simulink model "simple_FXTDiff_ANSFT"  (R2024b)
settings: Solver=ode4  StartTime=0.0  StopTime=15  FixedStep=0.01  RelTol=1e-3
model workspace (MAT data in the model file):
  roll = [0 0.5 0 -0.5 0 0.5]
  tra1 = [0 2 0 -2 0 2]
  tra2 = [0 2 2 2 2 0]
  tra3 = [0 0 2 2 2 2]
values from neighbouring files (symbols this model uses):
  F = 5    [assignment3.m]
undefined symbols (not defined in the file or in its folder): Light, MIL
libraries: dspobslib x7, simulink x5, robotcorelib x1, aerolibwind2 x1
settings Model: Creator=Adan Daniel  LastModifiedBy=danyy
settings OptimizationCC: ReuseModelBlockBuffer=off
settings RTWCC: GPUComputeCapability=3.5

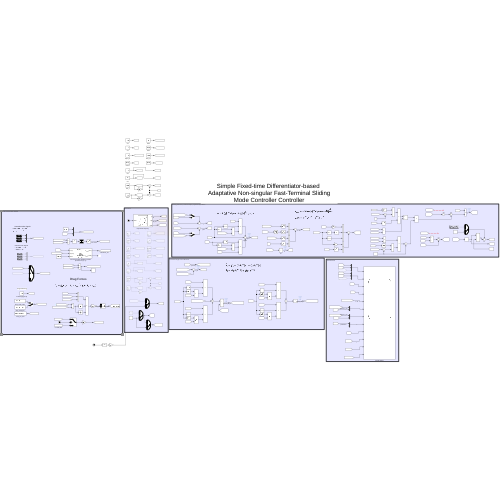
[thumbnail: Simulink's stored preview of the top-level diagram]
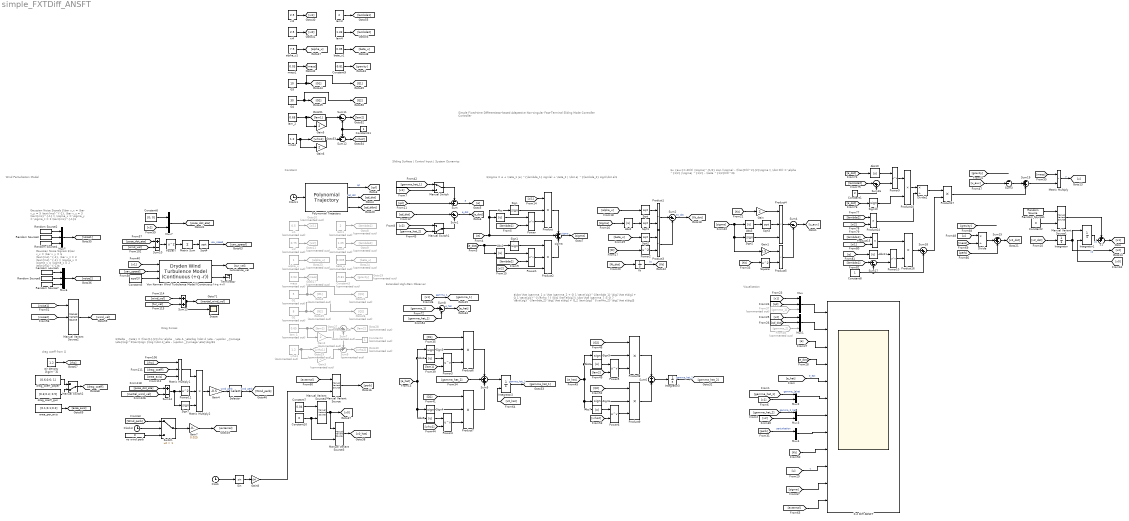
== system simple_FXTDiff_ANSFT ==
  note: Wind Perturbation Model
  note: Extended High-Gain Observer
  note: Sliding Surface | Control Input | System Dynamics
  note: Constant
  note: Visualization
  note: Simple Fixed-time Differentiator-based
      | Adaptative Non-singular Fast-Terminal Sliding Mode Controller Controller
  note: $\sigma = e + \zeta_1 |e| ^{\lambda_1} sign(e) + \zeta_2 | \dot e| ^{\lambda_2} sign(\dot e)$
  note: $u_{aux}=-2K(t) |\sigma|^{1/2} sign (\sigma) - \frac{K(t)^2}{2}\sigma \\ \dot K(t) = \alpha ^{1/2} |\sigma| ^{1/2} - \beta ^{1/2}K(t)^2$
  note: $\dot \hat \gamma_1 = \hat \gamma_2 + G_1 \text{sig}^{\lambda_1} \big[ \hat e\big] + Q_1 \text{sig}^{\varrho_1} \big[ \hat e\big] \\ \dot \hat \gamma_2 = G_2 \text{sig}^{\lambda_2} \big[ \hat e\big] + Q_2 \text{sig}^{\varrho_2} \big[ \hat e\big]$
  note: Gaussian Noise Signals
      | $\bar v_x = \bar v_y = 5 \text{ms}^{-1}, \bar v_z = 3 \text{ms}^{-1} \\ \sigma_x = \sigma_y = \sigma_z = 2 \text{ms}^{-1}$
  note: Gaussian Noise Signals
      | $\bar v_x = \bar v_y = 6 \text{ms}^{-1}, \bar v_z = 2 \text{ms}^{-1} \\ \sigma_x = \sigma_y = \sigma_z = 2 \text{ms}^{-1}$
  note: Drag Forces
  note: $\Delta _ {\eta} = \frac{1}{2}\rho \alpha _ \eta A _\eta\big (\dot d_\eta - \upsilon _{\omega \eta}\big)^2\text{sign }\big (\dot d_\eta - \upsilon _{\omega \eta}\big)$$
  note: drag coeff from []
  Abs{,1..7,10..11} (10 alike) : Abs  SaturateOnIntegerOverflow=off
  Clock : Clock
  Clock1 : Clock
  Clock3 : Clock
  Constant1 : Constant  Value=2
  Constant10 : Constant  Value=0
  Constant11 : Constant
  Constant2 : Constant  Value=0
  Constant3 : Constant  Commented=on  Value=-9.81
  Constant4 : Constant  Commented=on
  Constant5 : Constant  Value=eye(3)
  Constant6 : Constant  Value=[0; 0]
  Constant7 : Constant  Value=0.04
  Constant8 : Constant
  Constant9 : Constant  Value=-9.81
  Divide : Product  Inputs=*/
  Divide2 : Product  Inputs=*/
  From37 : From  Commented=on  GotoTag=gamma_1
  From38 : From  Commented=on  GotoTag=gamma_2
  Fxt Diff ANSFT : Scope  NumInputPorts=12
  G1 : Constant  Commented=on  Value=5
  G2 : Constant  Commented=on  Value=8
  G3 : Constant  Value=10
  G4 : Constant  Value=30
  Gain : Gain  Gain=2
  Gain1 : Gain  Gain=0.5
  Gain2 : Gain  Commented=on  Gain=2
  Gain3 : Gain  Commented=on  Gain=2
  Gain4 : Gain  Gain=-0.5
  Gain5 : Gain  Gain=2
  Gain6 : Gain  Gain=2
  Gain7 : Gain  Gain=0.025
  Gain8 : Gain  Gain=0.04
  Goto10 : Goto  Commented=on  GotoTag=xi1
  Goto11 : Goto  Commented=on  GotoTag=xi2
  Goto17 : Goto  Commented=on  GotoTag=mass
  Goto19 : Goto  Commented=on  GotoTag=gravity
  Goto2 : Goto  Commented=on  GotoTag=G1
  Goto22 : Goto  Commented=on  GotoTag=Q1
  Goto23 : Goto  Commented=on  GotoTag=alpha_u
  Goto24 : Goto  Commented=on  GotoTag=beta_u
  Goto25 : Goto  Commented=on  GotoTag=G2
  Goto26 : Goto  Commented=on  GotoTag=Q2
  Goto27 : Goto  Commented=on  GotoTag=lam1
  Goto28 : Goto  Commented=on  GotoTag=lam2
  Goto29 : Goto  Commented=on  GotoTag=vrho1
  Goto30 : Goto  Commented=on  GotoTag=vrho2
  Goto8 : Goto  Commented=on  GotoTag=lambda1
  Goto9 : Goto  Commented=on  GotoTag=lambda2
  Integrator : Integrator
  Integrator1 : Integrator  InitialConditionSource=external
  Integrator2 : Integrator  InitialConditionSource=external
  Integrator3 : Integrator
  Kt : Integrator
  Manual Variant Source{,1,3..4} (4 alike) : simulink/Signal Routing/Manual Variant Source  NumChoices=2  LabelModeActiveChoice=V_2
  Manual Variant Source2 : simulink/Signal Routing/Manual Variant Source  NumChoices=3  LabelModeActiveChoice=V_1
  Manual Switch : ManualSwitch
  Manual Switch1 : ManualSwitch  CurrentSetting=0
  Manual Switch2 : ManualSwitch  CurrentSetting=0
  Matrix Sum : Sum  Inputs=+
  Matrix Multiply : Product
  Matrix Multiply1 : Product  Inputs=3
  Matrix Multiply2 : Product  Inputs=3
  Mux{,1,5..6} (4 alike) : Mux  Inputs=3
  Mux{2..4,7} (4 alike) : Mux  Inputs=2
  Polynomial Trajectory : robotcorelib/Polynomial Trajectory  WaypointSource=Internal  Waypoints=[0, 0, 0.15, -0.15, 0.1, -0.1]*0  TimePoints=[0, 5, 10, 15, 20, 25]/5  TimeInterval=[ 1, 4 ]  Method=Cubic Polynomial  ParameterSource=Internal  VelocityBoundaryCondition=zeros( 1, 6 )  AccelerationBoundaryCondition=zeros( 2, 5 )  SimulateUsing=Interpreted execution
  Power{,1,3..6,9..10} (8 alike) : Math  Operator=pow
  Power11 : Math  Operator=square
  Power2 : Math  Operator=square
  Power7 : Math  Operator=square
  Product{,2,4,6..9} (7 alike) : Product  Inputs=3
  Product{1,3,5,10,14..17} (8 alike) : Product
  Random Source1 : dspobslib/Random Source  SrcType=Gaussian  NormMethod=Ziggurat  CltLength=12  MinVal=0  MaxVal=1  MeanVal=0.005  VarVal=0.001 * 0.001  RepMode=Repeatable  rawSeed=1  IsInherit=off  SampMode=Continuous  SampTime=0.01  SampFrame=1  DataType=Double  OutComplex=Real  OutputFrames=off
  Random Source2 : dspobslib/Random Source  SrcType=Gaussian  NormMethod=Ziggurat  CltLength=12  MinVal=0  MaxVal=1  MeanVal=5  VarVal=2  RepMode=Not repeatable  rawSeed=1  IsInherit=off  SampMode=Discrete  SampTime=1  SampFrame=1  DataType=Double  OutComplex=Real  OutputFrames=off
  Random Source3 : dspobslib/Random Source  SrcType=Gaussian  NormMethod=Ziggurat  CltLength=12  MinVal=0  MaxVal=1  MeanVal=5  VarVal=2  RepMode=Not repeatable  rawSeed=1  IsInherit=off  SampMode=Discrete  SampTime=1  SampFrame=1  DataType=Double  OutComplex=Real  OutputFrames=off
  Random Source4 : dspobslib/Random Source  SrcType=Gaussian  NormMethod=Ziggurat  CltLength=12  MinVal=0  MaxVal=1  MeanVal=3  VarVal=2  RepMode=Not repeatable  rawSeed=1  IsInherit=off  SampMode=Discrete  SampTime=1  SampFrame=1  DataType=Double  OutComplex=Real  OutputFrames=off
  Random Source5 : dspobslib/Random Source  SrcType=Gaussian  NormMethod=Ziggurat  CltLength=12  MinVal=0  MaxVal=1  MeanVal=6  VarVal=2  RepMode=Not repeatable  rawSeed=1  IsInherit=off  SampMode=Discrete  SampTime=1  SampFrame=1  DataType=Double  OutComplex=Real  OutputFrames=off
  Random Source6 : dspobslib/Random Source  SrcType=Gaussian  NormMethod=Ziggurat  CltLength=12  MinVal=0  MaxVal=1  MeanVal=6  VarVal=2  RepMode=Not repeatable  rawSeed=1  IsInherit=off  SampMode=Discrete  SampTime=1  SampFrame=1  DataType=Double  OutComplex=Real  OutputFrames=off
  Random Source7 : dspobslib/Random Source  SrcType=Gaussian  NormMethod=Ziggurat  CltLength=12  MinVal=0  MaxVal=1  MeanVal=2  VarVal=2  RepMode=Not repeatable  rawSeed=1  IsInherit=off  SampMode=Discrete  SampTime=1  SampFrame=1  DataType=Double  OutComplex=Real  OutputFrames=off
  Scope : Scope
  Selector : Selector  InputPortWidth=3  IndexOptions=Index vector (dialog)  Indices=[3]  OutputSizes=1
  Sign{,1..7,10} (9 alike) : Signum
  Sin : Trigonometry
  Sqrt{,1..4} (5 alike) : Sqrt
  Square : Math  Operator=square
  Sum : Sum  Inputs=-+|
  Sum{1..2,8,11,17} (5 alike) : Sum  Inputs=|+-
  Sum10 : Sum  Inputs=+-
  Sum12 : Sum  Inputs=-+|
  Sum13 : Sum
  Sum14 : Sum  Inputs=+-
  Sum15 : Sum  Inputs=+++
  Sum16 : Sum  Inputs=|-+
  Sum18 : Sum  Inputs=|++
  Sum19 : Sum  Inputs=+++
  Sum3 : Sum  Inputs=--|
  Sum4 : Sum  Inputs=|--
  Sum5 : Sum  Inputs=+++
  Sum6 : Sum  Inputs=+|+
  Sum7 : Sum  Commented=on  Inputs=|+-
  Sum9 : Sum  Commented=on  Inputs=-+|
  Switch : Switch  Criteria=u2 > Threshold  Threshold=1  SaturateOnIntegerOverflow=off  InputSameDT=off
  Terminator : Terminator
  Von Karman Wind Turbulence Model (Continuous (+q +r)) : aerolibwind2/Dryden Wind Turbulence Model  (Continuous (+q -r))  units=Metric (MKS)  spec=MIL-F-8785C  model=Continuous Von Karman (+q +r)  W20=15  Wdeg=0  TurbProb=10^-2 - Light  L_high=762  Wingspan=10  ts=0.1  Seed=[23341 23342 23343 23344]  T_on=on
      settings: LibrarySourceBlock=|
      | aerolibwind2/Von Karman Wind Turbulence Model
      | (Continuous (+q +r))
  air density [kg/m^3] : Constant  Value=1.2
  alpha_u : Constant  Commented=on
  alpha_u1 : Constant  Value=7.5
  area_per_axis : Constant  Value=[0.1;0.1;0.2]
  beta_u : Constant  Commented=on  Value=0.005
  beta_u1 : Constant  Value=0.05
  drag_coeff_gus : Constant  Value=[0.3;0.3; 0.5]
  drag_coeff_paper : Constant  Value=[0.6;0.6; 1]
  lam1 : Constant  Commented=on  Value=2
  lam2 : Constant  Commented=on  Value=1.25
  lam3 : Constant  Value=2
  lam4 : Constant  Value=1.33
  lam_1 : Constant  Commented=on  Value=0.65
  lam_2 : Constant  Value=0.68
  mass : Constant  Commented=on  Value=0.03
  mass1 : Constant  Value=0.03
  no wind perb : Constant  Value=0
  sigma : Sum  Inputs=+++
  vrho1 : Constant  Commented=on  Value=1.2
  vrho2 : Constant  Value=1.2
  x1 : Sum  Inputs=++|
  xi1 : Constant  Commented=on  Value=0.5
  xi2 : Constant  Commented=on  Value=0.75
  xi3 : Constant  Value=2.5
  xi4 : Constant  Value=2.5
  wires:
  Integrator/1 -> [x2], Integrator1/1  "x2"
  Sum1/1 -> [e_dot]  "e_dot"
  Mux/1 -> Fxt Diff ANSFT/1
  [x2_dot] -> Integrator/1
  Clock1/1 -> Polynomial Trajectory/1
  Polynomial Trajectory/3 -> [qd_ddot]
  [gamma_1] -> Sum8/1
  [gamma_hat_1] -> Sum8/2
  Sum8/1 -> [e_hat]  "e_hat"
  [e_hat] -> Fxt Diff ANSFT/5  "e_est"
  [gamma_hat_1] -> Mux2/1  "gamma_1_hat"
  [gamma_hat_2] -> Mux3/1  "gamma_2_hat"
  Mux2/1 -> Fxt Diff ANSFT/6
  [x1] -> Mux2/2
  Mux3/1 -> Fxt Diff ANSFT/7
  [x1] -> Manual Switch/2
  [x2] -> Manual Switch1/1
  [qd] -> Mux/2
  Polynomial Trajectory/1 -> [qd]  "qd"
  Polynomial Trajectory/2 -> [qd_dot]  "qd_dot"
  [qd] -> Sum/2
  [qd_dot] -> Sum1/1
  Sum/1 -> [e]  "e"
  lam1/1 -> Goto8/1
  lam2/1 -> Goto9/1
  xi1/1 -> Goto10/1
  xi2/1 -> Goto11/1
  [x1] -> Mux/1
  [qd_dot] -> Mux1/2
  [x2] -> Mux1/1
  Mux1/1 -> Fxt Diff ANSFT/2
  [e] -> Fxt Diff ANSFT/3
  [e_dot] -> Fxt Diff ANSFT/4
  [x1] -> [gamma_1]  "gamma_1"
  [x2] -> Mux3/2
  [perb] -> Mux4/1  "perturbation"
  Manual Variant Source/1 -> [perb]
  Mux4/1 -> Fxt Diff ANSFT/8
  mass/1 -> Goto17/1
  From37/1 -> Mux/3
  From38/1 -> Mux1/3
  Manual Switch/1 -> Sum/1
  Manual Switch1/1 -> Sum1/2
  [gamma_hat_2] -> Manual Switch1/2
  [gamma_hat_1] -> Manual Switch/1
  Constant3/1 -> Goto19/1
  [Kt] -> Fxt Diff ANSFT/9
  [u] -> Fxt Diff ANSFT/10  "u"
  [u] -> Divide/1
  [e] -> sigma/2, Abs/1, Sign/1
  Abs/1 -> Power/1
  [lambda1] -> Power/2
  Power/1 -> Product/3
  Sign/1 -> Product/2
  sigma/1 -> [sigma]  "sigma"
  Power1/1 -> Product2/2
  [e_dot] -> Abs1/1, Sign1/1
  [lambda2] -> Power1/2
  Abs1/1 -> Power1/1
  Sign1/1 -> Product2/1
  Product2/1 -> sigma/3
  Product/1 -> sigma/1
  [xi1] -> Product/1
  [xi2] -> Product2/3
  beta_u/1 -> Goto24/1
  alpha_u/1 -> Goto23/1
  [Kt] -> Power2/1
  [alpha_u] -> Sqrt/1
  [sigma] -> Abs2/1
  Abs2/1 -> Sqrt1/1
  Sqrt1/1 -> Product1/2
  Power2/1 -> Product3/2
  [beta_u] -> Sqrt2/1
  Sqrt/1 -> Product1/1
  Product3/1 -> Sum2/2
  Product1/1 -> Sum2/1
  Sqrt2/1 -> Product3/1
  Sum2/1 -> [Kt_dot]  "Kt_dot"
  [Kt_dot] -> Kt/1
  Kt/1 -> [Kt]  "kt"
  Sqrt3/1 -> Product4/2
  Product4/1 -> Sum4/1
  Abs3/1 -> Sqrt3/1
  [sigma] -> Abs3/1, Sign2/1, Gain1/1
  Gain/1 -> Product4/1
  [Kt] -> Gain/1
  Sign2/1 -> Product4/3
  [Kt] -> Square/1
  Square/1 -> Product5/2
  Gain1/1 -> Product5/1
  Product5/1 -> Sum4/2
  Sum4/1 -> [u_aux]
  Matrix Multiply/1 -> [u]  "u"
  Sum15/1 -> [x2_dot]
  [sigma] -> Fxt Diff ANSFT/11
  [mass] -> Divide/2
  Divide/1 -> Sum15/2
  [perb] -> Sum15/3
  [gravity] -> ?
  [mass] -> Matrix Multiply/1
  [u_aux] -> Sum3/2
  [e_dot] -> Abs10/1
  Sum16/1 -> Power9/2
  Sign10/1 -> Product10/2
  Abs10/1 -> Power9/1
  Product14/1 -> Divide2/2
  Constant1/1 -> Sum16/2
  [lambda2] -> Sum16/1
  Power9/1 -> Product10/1
  [lambda2] -> Product14/1
  [e_dot] -> Sign10/1
  Product10/1 -> Divide2/1
  [xi2] -> Product14/2
  Product15/1 -> Product16/1
  Product16/1 -> Sum18/1
  Power10/1 -> Product16/2
  Constant8/1 -> Sum18/2, Sum17/2
  [xi1] -> Product15/2
  [lambda1] -> Product15/1
  Abs11/1 -> Power10/1
  [lambda1] -> Sum17/1
  [e] -> Abs11/1
  Sum17/1 -> Power10/2
  Divide2/1 -> Product17/1
  Sum18/1 -> Product17/2
  Sum19/1 -> Matrix Multiply/2
  Sum3/1 -> Sum19/2
  Product17/1 -> Sum19/3
  Sum5/1 -> Integrator2/1
  Sign6/1 -> Product9/2
  Power5/1 -> Product8/3
  Power6/1 -> Product9/3
  [Q2] -> Product9/1
  [G2] -> Product8/1
  Power4/1 -> Product7/3
  [vrho2] -> Power6/2
  Sign5/1 -> Product8/2
  Product7/1 -> Sum5/3
  [Q1] -> Product7/1
  Integrator3/1 -> [gamma_hat_2]  "gamma_hat_2"
  Product8/1 -> Sum6/1
  [gamma_hat_2] -> Sum5/2
  [lam2] -> Power5/2
  [lam1] -> Power3/2
  Abs4/1 -> Power3/1
  Power3/1 -> Product6/3
  [e_hat] -> Sign3/1, Abs4/1, Abs5/1, Sign4/1
  [G1] -> Product6/1
  Integrator2/1 -> [gamma_hat_1]  "gamma_hat_1"
  Product6/1 -> Sum5/1
  Abs7/1 -> Power6/1
  Sign4/1 -> Product7/2
  Abs5/1 -> Power4/1
  Abs6/1 -> Power5/1
  [vrho1] -> Power4/2
  Product9/1 -> Sum6/2
  Sign3/1 -> Product6/2
  Sum6/1 -> Integrator3/1
  [e_hat] -> Sign5/1, Abs6/1, Abs7/1, Sign6/1
  G2/1 -> Goto26/1, Goto25/1
  lam_1/1 -> Gain2/1, Goto27/1
  vrho1/1 -> Gain3/1, Goto29/1
  G1/1 -> Goto22/1, Goto2/1
  [gravity] -> ?
  Constant2/1 -> Manual Variant Source1/2
  Random Source1/1 -> Manual Variant Source1/1
  Integrator1/1 -> x1/2  "x1"
  x1/1 -> [x1]
  Manual Variant Source1/1 -> x1/1
  Gain2/1 -> Sum7/1
  Sum7/1 -> Goto28/1
  Constant4/1 -> Sum7/2, Sum9/1
  Gain3/1 -> Sum9/2
  Sum9/1 -> Goto30/1
  Constant5/1 -> Von Karman Wind Turbulence Model (Continuous (+q +r))/3
  [x1] -> Von Karman Wind Turbulence Model (Continuous (+q +r))/1
  Von Karman Wind Turbulence Model (Continuous (+q +r))/1 -> [tur_vel]
  [tur_vel] -> Sum13/2
  Sum13/1 -> Scope/1, [inertial_wind_vel]
  [wind_vel] -> Sum13/1
  Random Source4/1 -> Mux5/3
  Mux5/1 -> [noise1]
  Random Source6/1 -> Mux6/2
  Random Source7/1 -> Mux6/3
  Mux6/1 -> [noise2]
  Random Source5/1 -> Mux6/1
  [noise2] -> Manual Variant Source2/2
  Manual Variant Source2/1 -> [wind_vel]
  Random Source3/1 -> Mux5/2
  Random Source2/1 -> Mux5/1
  [noise1] -> Manual Variant Source2/1
  [wind_vel] -> Sum10/2
  Sqrt4/1 -> [uav_speed]  "uav_speed"
  Mux7/1 -> [pose_dot_eta]
  Power7/1 -> Matrix Sum/1
  Sum10/1 -> Power7/1
  Matrix Sum/1 -> Sqrt4/1
  [uav_speed] -> Von Karman Wind Turbulence Model (Continuous (+q +r))/2
  [x2] -> Mux7/2
  Constant6/1 -> Mux7/1
  [drag_coeff] -> Matrix Multiply1/2
  Matrix Multiply2/1 -> Gain4/1
  [rho] -> Matrix Multiply1/1
  drag_coeff_paper/1 -> Manual Switch2/1
  Sign7/1 -> Matrix Multiply2/3
  Power11/1 -> Matrix Multiply2/2
  drag_coeff_gus/1 -> Manual Switch2/2
  air density [kg/m^3]/1 -> [rho]
  Matrix Multiply1/1 -> Matrix Multiply2/1
  Gain4/1 -> Selector/1  "wind_perb"
  area_per_axis/1 -> [area_axis]
  [pose_dot_eta] -> Sum14/1
  Sum14/1 -> Sign7/1, Power11/1
  [inertial_wind_vel] -> Sum14/2
  [area_axis] -> Matrix Multiply1/3
  Manual Switch2/1 -> [drag_coeff]
  Sin/1 -> Gain8/1
  [external] -> Manual Variant Source/1
  Selector/1 -> [Wind_perb]  "wind_perb"
  [pose_dot_eta] -> Sum10/1
  Von Karman Wind Turbulence Model (Continuous (+q +r))/2 -> Terminator/1
  [external] -> Fxt Diff ANSFT/12
  [x0] -> Integrator1/2
  [x0_hat] -> Integrator2/2
  Manual Variant Source3/1 -> [x0_hat]
  Constant10/1 -> Manual Variant Source3/2, Manual Variant Source4/2
  Manual Variant Source4/1 -> Manual Variant Source3/1, [x0]
  Constant7/1 -> Manual Variant Source4/1
  no wind perb/1 -> Switch/3
  Clock3/1 -> Switch/2
  [Wind_perb] -> Switch/1
  Switch/1 -> Gain7/1
  Gain5/1 -> Sum11/1
  xi4/1 -> [xi2]
  vrho2/1 -> Gain6/1, [vrho1]
  Sum12/1 -> [vrho2]
  lam4/1 -> [lambda2]
  lam_2/1 -> Gain5/1, [lam1]
  alpha_u1/1 -> [alpha_u]
  G4/1 -> [Q2], [G2]
  xi3/1 -> [xi1]
  mass1/1 -> [mass]
  Constant11/1 -> Sum11/2, Sum12/1
  Gain6/1 -> Sum12/2
  beta_u1/1 -> [beta_u]
  lam3/1 -> [lambda1]
  Sum11/1 -> [lam2]
  Constant9/1 -> [gravity]
  G3/1 -> [Q1], [G1]
  Gain7/1 -> [external]
  Clock/1 -> Sin/1
  Gain8/1 -> Manual Variant Source/2
